simulink model "husky_sim - Copy"  (R2019b)
settings: Solver=ode4  StartTime=0.0  StopTime=3  FixedStep=0.006  RelTol=1e-3
InitFcn:
  | init_model;
values from neighbouring files (symbols this model uses):
  m = getfield(leg,'mass')    [dynamic_test.m]    (also in pen_init.m = link2.mass; test.mat = 2.2337)
  q_BL_K0 = initial_angle(12)    [func_params_ext.m]
  q_BR_K0 = initial_angle(9)    [func_params_ext.m]
  q_FL_K0 = initial_angle(6)    [func_params_ext.m]
undefined symbols (not defined in the file or in its folder): body, femur_left, femur_right, hip_left, hip_right, link_left, link_right, tarsus_left, tarsus_right, tibia_left, tibia_right, X, Y, Z
libraries: sm_lib x206, nesl_utility x56, dspsigops x7, Contact_Forces_Lib x4, simulink x2
(part 5 of 6)

== system husky_sim - Copy/Husky_simulator/robot_body/Leg_RL/tibia_rl ==
  Inertia : sm_lib/Body Elements/Inertia  InertiaType=Custom  Mass=tibia_left.mass  MassUnits=kg  CenterOfMass=[0, 0, 0]  CenterOfMassUnits=m  MomentsOfInertia=tibia_left.MomentsofInertia  MomentsOfInertiaUnits=kg*m^2  ProductsOfInertia=tibia_left.ProductsofInertia  ProductsOfInertiaUnits=kg*m^2  GraphicType=None  MarkerShape=Inertia  MarkerSize=20  GraphicVisPropType=SimpleVisualProperties  GraphicDiffuseColor=[0.5 0.5 0.5]  GraphicSpecularColor=[0.5 0.5 0.5 1.0]  GraphicAmbientColor=[0.15 0.15 0.15 1.0]  GraphicEmissiveColor=[0.0 0.0 0.0 1.0]  GraphicShininess=75  GraphicOpacity=1.0
  InertiaOriginTransform : sm_lib/Frames and Transforms/Rigid Transform  TranslationMethod=Cartesian  TranslationStandardOffset=0  TranslationLengthUnit=m  TranslationStandardAxis=+Z  TranslationCartesianOffset=[-0.10575, 0.0039831, 1.084e-05]  TranslationROffset=0  TranslationROffsetUnits=m  TranslationZOffset=0  TranslationZOffsetUnits=m  TranslationThetaOffset=0  TranslationThetaOffsetUnits=deg  RotationMethod=RotationSequence  RotationAngleUnits=deg  RotationStandardAxis=+Z  RotationAngle=0.0  RotationArbitraryAxis=[0 0 1]  FollAlignAxisA=+X  BaseAlignAxisA=+Y  FollAlignAxisB=+Y  BaseAlignAxisB=+Z  RotationSequenceAxes=BaseAxes  RotationSequence=XYZ  RotationSequenceAngles=[0, 0, 0]  RotationSequenceAnglesUnits=rad  RotationMatrix=[1 0 0; 0 1 0; 0 0 1]
  ReferenceFrame : sm_lib/Frames and Transforms/Reference Frame
  Visual : sm_lib/Body Elements/File Solid  ExtGeomFileName=husky/meshes/tibia_rl.STL  UnitType=Custom  ExtGeomFileUnits=m  StepReaderType=HEX  ExportEntireGeometry=off  InertiaType=Custom  Mass=0  MassUnits=kg  CenterOfMass=[0, 0, 0]  CenterOfMassUnits=m  MomentsOfInertia=[0, 0, 0]  MomentsOfInertiaUnits=kg*m^2  ProductsOfInertia=[0, 0, 0]  ProductsOfInertiaUnits=kg*m^2  BasedOnType=DensityFromFile  Density=1000  DensityUnits=kg/m^3  DoExposeReferenceFrame=on  SerializedFrames=<Frames/>  GraphicType=FromGeometry  MarkerShape=Sphere  MarkerSize=10  GraphicVisPropType=SimpleVisualProperties  GraphicDiffuseColor=[0, 0, 1]  GraphicSpecularColor=[0.5 0.5 0.5 1.0]  GraphicAmbientColor=[0.15 0.15 0.15 1.0]  GraphicEmissiveColor=[0.0 0.0 0.0 1.0]  GraphicShininess=75  GraphicOpacity=1
  VisualOriginTransform : sm_lib/Frames and Transforms/Rigid Transform  TranslationMethod=Cartesian  TranslationStandardOffset=0  TranslationLengthUnit=m  TranslationStandardAxis=+Z  TranslationCartesianOffset=[0, 0, 0]  TranslationROffset=0  TranslationROffsetUnits=m  TranslationZOffset=0  TranslationZOffsetUnits=m  TranslationThetaOffset=0  TranslationThetaOffsetUnits=deg  RotationMethod=RotationSequence  RotationAngleUnits=deg  RotationStandardAxis=+Z  RotationAngle=0.0  RotationArbitraryAxis=[0 0 1]  FollAlignAxisA=+X  BaseAlignAxisA=+Y  FollAlignAxisB=+Y  BaseAlignAxisB=+Z  RotationSequenceAxes=BaseAxes  RotationSequence=XYZ  RotationSequenceAngles=[0, 0, 0]  RotationSequenceAnglesUnits=rad  RotationMatrix=[1 0 0; 0 1 0; 0 0 1]
  ankle_rl_AxisTransform : sm_lib/Frames and Transforms/Rigid Transform  TranslationMethod=Cartesian  TranslationStandardOffset=0  TranslationLengthUnit=m  TranslationStandardAxis=+Z  TranslationCartesianOffset=[0, 0, 0]  TranslationROffset=0  TranslationROffsetUnits=m  TranslationZOffset=0  TranslationZOffsetUnits=m  TranslationThetaOffset=0  TranslationThetaOffsetUnits=deg  RotationMethod=ArbitraryAxis  RotationAngleUnits=rad  RotationStandardAxis=+Z  RotationAngle=-1.570796326794897  RotationArbitraryAxis=[-1, 0, 0]  FollAlignAxisA=+X  BaseAlignAxisA=+Y  FollAlignAxisB=+Y  BaseAlignAxisB=+Z  RotationSequenceAxes=FollowerAxes  RotationSequence=XYX  RotationSequenceAngles=[0 0 0]  RotationSequenceAnglesUnits=deg  RotationMatrix=[1 0 0; 0 1 0; 0 0 1]
  ankle_rl_OriginTransform : sm_lib/Frames and Transforms/Rigid Transform  TranslationMethod=Cartesian  TranslationStandardOffset=0  TranslationLengthUnit=m  TranslationStandardAxis=+Z  TranslationCartesianOffset=[-0.333, 0.0075, 0]  TranslationROffset=0  TranslationROffsetUnits=m  TranslationZOffset=0  TranslationZOffsetUnits=m  TranslationThetaOffset=0  TranslationThetaOffsetUnits=deg  RotationMethod=RotationSequence  RotationAngleUnits=deg  RotationStandardAxis=+Z  RotationAngle=0.0  RotationArbitraryAxis=[0 0 1]  FollAlignAxisA=+X  BaseAlignAxisA=+Y  FollAlignAxisB=+Y  BaseAlignAxisB=+Z  RotationSequenceAxes=BaseAxes  RotationSequence=XYZ  RotationSequenceAngles=[0, 0, 0]  RotationSequenceAnglesUnits=rad  RotationMatrix=[1 0 0; 0 1 0; 0 0 1]
  knee_rl_AxisInvTransform : sm_lib/Frames and Transforms/Rigid Transform  TranslationMethod=Cartesian  TranslationStandardOffset=0  TranslationLengthUnit=m  TranslationStandardAxis=+Z  TranslationCartesianOffset=[0, 0, 0]  TranslationROffset=0  TranslationROffsetUnits=m  TranslationZOffset=0  TranslationZOffsetUnits=m  TranslationThetaOffset=0  TranslationThetaOffsetUnits=deg  RotationMethod=ArbitraryAxis  RotationAngleUnits=rad  RotationStandardAxis=+Z  RotationAngle=1.570796326794897  RotationArbitraryAxis=[1, 0, 0]  FollAlignAxisA=+X  BaseAlignAxisA=+Y  FollAlignAxisB=+Y  BaseAlignAxisB=+Z  RotationSequenceAxes=FollowerAxes  RotationSequence=XYX  RotationSequenceAngles=[0 0 0]  RotationSequenceAnglesUnits=deg  RotationMatrix=[1 0 0; 0 1 0; 0 0 1]
  F : PMIOPort  Side=Left
  F1 : PMIOPort  Port=2  Side=Right
  connections:
  Inertia/RConn1 -- InertiaOriginTransform/RConn1
  ankle_rl_OriginTransform/LConn1 -- knee_rl_AxisInvTransform/LConn1 -- InertiaOriginTransform/LConn1 -- ReferenceFrame/RConn1 -- VisualOriginTransform/LConn1
  Visual/RConn1 -- VisualOriginTransform/RConn1
  ankle_rl_AxisTransform/RConn1 -- F1/RConn1
  ankle_rl_AxisTransform/LConn1 -- ankle_rl_OriginTransform/RConn1
  knee_rl_AxisInvTransform/RConn1 -- F/RConn1

== system husky_sim - Copy/Husky_simulator/robot_body/Leg_RR/femur_rr ==
  Inertia : sm_lib/Body Elements/Inertia  InertiaType=Custom  Mass=femur_right.mass  MassUnits=kg  CenterOfMass=[0, 0, 0]  CenterOfMassUnits=m  MomentsOfInertia=femur_right.MomentsofInertia  MomentsOfInertiaUnits=kg*m^2  ProductsOfInertia=femur_right.ProductsofInertia  ProductsOfInertiaUnits=kg*m^2  GraphicType=None  MarkerShape=Inertia  MarkerSize=20  GraphicVisPropType=SimpleVisualProperties  GraphicDiffuseColor=[0.5 0.5 0.5]  GraphicSpecularColor=[0.5 0.5 0.5 1.0]  GraphicAmbientColor=[0.15 0.15 0.15 1.0]  GraphicEmissiveColor=[0.0 0.0 0.0 1.0]  GraphicShininess=75  GraphicOpacity=1.0
  InertiaOriginTransform : sm_lib/Frames and Transforms/Rigid Transform  TranslationMethod=Cartesian  TranslationStandardOffset=0  TranslationLengthUnit=m  TranslationStandardAxis=+Z  TranslationCartesianOffset=[2.704e-07, -0.036112, -0.082829]  TranslationROffset=0  TranslationROffsetUnits=m  TranslationZOffset=0  TranslationZOffsetUnits=m  TranslationThetaOffset=0  TranslationThetaOffsetUnits=deg  RotationMethod=RotationSequence  RotationAngleUnits=deg  RotationStandardAxis=+Z  RotationAngle=0.0  RotationArbitraryAxis=[0 0 1]  FollAlignAxisA=+X  BaseAlignAxisA=+Y  FollAlignAxisB=+Y  BaseAlignAxisB=+Z  RotationSequenceAxes=BaseAxes  RotationSequence=XYZ  RotationSequenceAngles=[0, 0, 0]  RotationSequenceAnglesUnits=rad  RotationMatrix=[1 0 0; 0 1 0; 0 0 1]
  ReferenceFrame : sm_lib/Frames and Transforms/Reference Frame
  Visual : sm_lib/Body Elements/File Solid  ExtGeomFileName=husky/meshes/femur_rr.STL  UnitType=Custom  ExtGeomFileUnits=m  StepReaderType=HEX  ExportEntireGeometry=off  InertiaType=Custom  Mass=0  MassUnits=kg  CenterOfMass=[0, 0, 0]  CenterOfMassUnits=m  MomentsOfInertia=[0, 0, 0]  MomentsOfInertiaUnits=kg*m^2  ProductsOfInertia=[0, 0, 0]  ProductsOfInertiaUnits=kg*m^2  BasedOnType=DensityFromFile  Density=1000  DensityUnits=kg/m^3  DoExposeReferenceFrame=on  SerializedFrames=<Frames/>  GraphicType=FromGeometry  MarkerShape=Sphere  MarkerSize=10  GraphicVisPropType=SimpleVisualProperties  GraphicDiffuseColor=[0, 1, 0]  GraphicSpecularColor=[0.5 0.5 0.5 1.0]  GraphicAmbientColor=[0.15 0.15 0.15 1.0]  GraphicEmissiveColor=[0.0 0.0 0.0 1.0]  GraphicShininess=75  GraphicOpacity=1
  VisualOriginTransform : sm_lib/Frames and Transforms/Rigid Transform  TranslationMethod=Cartesian  TranslationStandardOffset=0  TranslationLengthUnit=m  TranslationStandardAxis=+Z  TranslationCartesianOffset=[0, 0, 0]  TranslationROffset=0  TranslationROffsetUnits=m  TranslationZOffset=0  TranslationZOffsetUnits=m  TranslationThetaOffset=0  TranslationThetaOffsetUnits=deg  RotationMethod=RotationSequence  RotationAngleUnits=deg  RotationStandardAxis=+Z  RotationAngle=0.0  RotationArbitraryAxis=[0 0 1]  FollAlignAxisA=+X  BaseAlignAxisA=+Y  FollAlignAxisB=+Y  BaseAlignAxisB=+Z  RotationSequenceAxes=BaseAxes  RotationSequence=XYZ  RotationSequenceAngles=[0, 0, 0]  RotationSequenceAnglesUnits=rad  RotationMatrix=[1 0 0; 0 1 0; 0 0 1]
  hip_rr_ex_AxisInvTransform : sm_lib/Frames and Transforms/Rigid Transform  TranslationMethod=Cartesian  TranslationStandardOffset=0  TranslationLengthUnit=m  TranslationStandardAxis=+Z  TranslationCartesianOffset=[0, 0, 0]  TranslationROffset=0  TranslationROffsetUnits=m  TranslationZOffset=0  TranslationZOffsetUnits=m  TranslationThetaOffset=0  TranslationThetaOffsetUnits=deg  RotationMethod=ArbitraryAxis  RotationAngleUnits=rad  RotationStandardAxis=+Z  RotationAngle=1.570796326794897  RotationArbitraryAxis=[1, 0, 0]  FollAlignAxisA=+X  BaseAlignAxisA=+Y  FollAlignAxisB=+Y  BaseAlignAxisB=+Z  RotationSequenceAxes=FollowerAxes  RotationSequence=XYX  RotationSequenceAngles=[0 0 0]  RotationSequenceAnglesUnits=deg  RotationMatrix=[1 0 0; 0 1 0; 0 0 1]
  knee_rr_AxisTransform : sm_lib/Frames and Transforms/Rigid Transform  TranslationMethod=Cartesian  TranslationStandardOffset=0  TranslationLengthUnit=m  TranslationStandardAxis=+Z  TranslationCartesianOffset=[0, 0, 0]  TranslationROffset=0  TranslationROffsetUnits=m  TranslationZOffset=0  TranslationZOffsetUnits=m  TranslationThetaOffset=0  TranslationThetaOffsetUnits=deg  RotationMethod=ArbitraryAxis  RotationAngleUnits=rad  RotationStandardAxis=+Z  RotationAngle=1.570796326794897  RotationArbitraryAxis=[-1, 0, 0]  FollAlignAxisA=+X  BaseAlignAxisA=+Y  FollAlignAxisB=+Y  BaseAlignAxisB=+Z  RotationSequenceAxes=FollowerAxes  RotationSequence=XYX  RotationSequenceAngles=[0 0 0]  RotationSequenceAnglesUnits=deg  RotationMatrix=[1 0 0; 0 1 0; 0 0 1]
  knee_rr_OriginTransform : sm_lib/Frames and Transforms/Rigid Transform  TranslationMethod=Cartesian  TranslationStandardOffset=0  TranslationLengthUnit=m  TranslationStandardAxis=+Z  TranslationCartesianOffset=[0, 0, -0.158]  TranslationROffset=0  TranslationROffsetUnits=m  TranslationZOffset=0  TranslationZOffsetUnits=m  TranslationThetaOffset=0  TranslationThetaOffsetUnits=deg  RotationMethod=RotationSequence  RotationAngleUnits=deg  RotationStandardAxis=+Z  RotationAngle=0.0  RotationArbitraryAxis=[0 0 1]  FollAlignAxisA=+X  BaseAlignAxisA=+Y  FollAlignAxisB=+Y  BaseAlignAxisB=+Z  RotationSequenceAxes=BaseAxes  RotationSequence=XYZ  RotationSequenceAngles=[0, 0, 0]  RotationSequenceAnglesUnits=rad  RotationMatrix=[1 0 0; 0 1 0; 0 0 1]
  F : PMIOPort  Side=Left
  F1 : PMIOPort  Port=2  Side=Right
  connections:
  Inertia/RConn1 -- InertiaOriginTransform/RConn1
  InertiaOriginTransform/LConn1 -- hip_rr_ex_AxisInvTransform/LConn1 -- knee_rr_OriginTransform/LConn1 -- VisualOriginTransform/LConn1 -- ReferenceFrame/RConn1
  Visual/RConn1 -- VisualOriginTransform/RConn1
  hip_rr_ex_AxisInvTransform/RConn1 -- F/RConn1
  knee_rr_AxisTransform/RConn1 -- F1/RConn1
  knee_rr_AxisTransform/LConn1 -- knee_rr_OriginTransform/RConn1

== system husky_sim - Copy/Husky_simulator/robot_body/Leg_RR/hip_rr ==
  Inertia : sm_lib/Body Elements/Inertia  InertiaType=Custom  Mass=hip_right.mass  MassUnits=kg  CenterOfMass=[0,0,0]  CenterOfMassUnits=m  MomentsOfInertia=hip_right.MomentsofInertia  MomentsOfInertiaUnits=kg*m^2  ProductsOfInertia=hip_right.ProductsofInertia  ProductsOfInertiaUnits=kg*m^2  GraphicType=None  MarkerShape=Inertia  MarkerSize=20  GraphicVisPropType=SimpleVisualProperties  GraphicDiffuseColor=[0.5 0.5 0.5]  GraphicSpecularColor=[0.5 0.5 0.5 1.0]  GraphicAmbientColor=[0.15 0.15 0.15 1.0]  GraphicEmissiveColor=[0.0 0.0 0.0 1.0]  GraphicShininess=75  GraphicOpacity=1.0
  InertiaOriginTransform : sm_lib/Frames and Transforms/Rigid Transform  TranslationMethod=Cartesian  TranslationStandardOffset=0  TranslationLengthUnit=m  TranslationStandardAxis=+Z  TranslationCartesianOffset=[0.024751, 0.0025459, 6.0284e-05]  TranslationROffset=0  TranslationROffsetUnits=m  TranslationZOffset=0  TranslationZOffsetUnits=m  TranslationThetaOffset=0  TranslationThetaOffsetUnits=deg  RotationMethod=RotationSequence  RotationAngleUnits=deg  RotationStandardAxis=+Z  RotationAngle=0.0  RotationArbitraryAxis=[0 0 1]  FollAlignAxisA=+X  BaseAlignAxisA=+Y  FollAlignAxisB=+Y  BaseAlignAxisB=+Z  RotationSequenceAxes=BaseAxes  RotationSequence=XYZ  RotationSequenceAngles=[0, 0, 0]  RotationSequenceAnglesUnits=rad  RotationMatrix=[1 0 0; 0 1 0; 0 0 1]
  ReferenceFrame : sm_lib/Frames and Transforms/Reference Frame
  Visual : sm_lib/Body Elements/File Solid  ExtGeomFileName=husky/meshes/hip_rr.STL  UnitType=Custom  ExtGeomFileUnits=m  StepReaderType=HEX  ExportEntireGeometry=off  InertiaType=Custom  Mass=0  MassUnits=kg  CenterOfMass=[0, 0, 0]  CenterOfMassUnits=m  MomentsOfInertia=[0, 0, 0]  MomentsOfInertiaUnits=kg*m^2  ProductsOfInertia=[0, 0, 0]  ProductsOfInertiaUnits=kg*m^2  BasedOnType=DensityFromFile  Density=1000  DensityUnits=kg/m^3  DoExposeReferenceFrame=on  SerializedFrames=<Frames/>  GraphicType=FromGeometry  MarkerShape=Sphere  MarkerSize=10  GraphicVisPropType=SimpleVisualProperties  GraphicDiffuseColor=[1, 0, 0]  GraphicSpecularColor=[0.5 0.5 0.5 1.0]  GraphicAmbientColor=[0.15 0.15 0.15 1.0]  GraphicEmissiveColor=[0.0 0.0 0.0 1.0]  GraphicShininess=75  GraphicOpacity=1
  VisualOriginTransform : sm_lib/Frames and Transforms/Rigid Transform  TranslationMethod=Cartesian  TranslationStandardOffset=0  TranslationLengthUnit=m  TranslationStandardAxis=+Z  TranslationCartesianOffset=[0, 0, 0]  TranslationROffset=0  TranslationROffsetUnits=m  TranslationZOffset=0  TranslationZOffsetUnits=m  TranslationThetaOffset=0  TranslationThetaOffsetUnits=deg  RotationMethod=RotationSequence  RotationAngleUnits=deg  RotationStandardAxis=+Z  RotationAngle=0.0  RotationArbitraryAxis=[0 0 1]  FollAlignAxisA=+X  BaseAlignAxisA=+Y  FollAlignAxisB=+Y  BaseAlignAxisB=+Z  RotationSequenceAxes=BaseAxes  RotationSequence=XYZ  RotationSequenceAngles=[0, 0, 0]  RotationSequenceAnglesUnits=rad  RotationMatrix=[1 0 0; 0 1 0; 0 0 1]
  hip_rr_ab_AxisInvTransform : sm_lib/Frames and Transforms/Rigid Transform  TranslationMethod=Cartesian  TranslationStandardOffset=0  TranslationLengthUnit=m  TranslationStandardAxis=+Z  TranslationCartesianOffset=[0, 0, 0]  TranslationROffset=0  TranslationROffsetUnits=m  TranslationZOffset=0  TranslationZOffsetUnits=m  TranslationThetaOffset=0  TranslationThetaOffsetUnits=deg  RotationMethod=ArbitraryAxis  RotationAngleUnits=rad  RotationStandardAxis=+Z  RotationAngle=1.570796326794897  RotationArbitraryAxis=[-0, -1, 0]  FollAlignAxisA=+X  BaseAlignAxisA=+Y  FollAlignAxisB=+Y  BaseAlignAxisB=+Z  RotationSequenceAxes=FollowerAxes  RotationSequence=XYX  RotationSequenceAngles=[0 0 0]  RotationSequenceAnglesUnits=deg  RotationMatrix=[1 0 0; 0 1 0; 0 0 1]
  hip_rr_ex_AxisTransform : sm_lib/Frames and Transforms/Rigid Transform  TranslationMethod=Cartesian  TranslationStandardOffset=0  TranslationLengthUnit=m  TranslationStandardAxis=+Z  TranslationCartesianOffset=[0, 0, 0]  TranslationROffset=0  TranslationROffsetUnits=m  TranslationZOffset=0  TranslationZOffsetUnits=m  TranslationThetaOffset=0  TranslationThetaOffsetUnits=deg  RotationMethod=ArbitraryAxis  RotationAngleUnits=rad  RotationStandardAxis=+Z  RotationAngle=1.570796326794897  RotationArbitraryAxis=[1, 0, 0]  FollAlignAxisA=+X  BaseAlignAxisA=+Y  FollAlignAxisB=+Y  BaseAlignAxisB=+Z  RotationSequenceAxes=FollowerAxes  RotationSequence=XYX  RotationSequenceAngles=[0 0 0]  RotationSequenceAnglesUnits=deg  RotationMatrix=[1 0 0; 0 1 0; 0 0 1]
  hip_rr_ex_OriginTransform : sm_lib/Frames and Transforms/Rigid Transform  TranslationMethod=Cartesian  TranslationStandardOffset=0  TranslationLengthUnit=m  TranslationStandardAxis=+Z  TranslationCartesianOffset=[0.053, 0.007, 0]  TranslationROffset=0  TranslationROffsetUnits=m  TranslationZOffset=0  TranslationZOffsetUnits=m  TranslationThetaOffset=0  TranslationThetaOffsetUnits=deg  RotationMethod=RotationSequence  RotationAngleUnits=deg  RotationStandardAxis=+Z  RotationAngle=0.0  RotationArbitraryAxis=[0 0 1]  FollAlignAxisA=+X  BaseAlignAxisA=+Y  FollAlignAxisB=+Y  BaseAlignAxisB=+Z  RotationSequenceAxes=BaseAxes  RotationSequence=XYZ  RotationSequenceAngles=[0, 0, 0]  RotationSequenceAnglesUnits=rad  RotationMatrix=[1 0 0; 0 1 0; 0 0 1]
  F : PMIOPort  Side=Left
  F1 : PMIOPort  Port=2  Side=Right
  connections:
  Inertia/RConn1 -- InertiaOriginTransform/RConn1
  hip_rr_ab_AxisInvTransform/LConn1 -- hip_rr_ex_OriginTransform/LConn1 -- InertiaOriginTransform/LConn1 -- ReferenceFrame/RConn1 -- VisualOriginTransform/LConn1
  Visual/RConn1 -- VisualOriginTransform/RConn1
  hip_rr_ab_AxisInvTransform/RConn1 -- F/RConn1
  hip_rr_ex_AxisTransform/RConn1 -- F1/RConn1
  hip_rr_ex_AxisTransform/LConn1 -- hip_rr_ex_OriginTransform/RConn1

== system husky_sim - Copy/Husky_simulator/robot_body/Leg_RR/link_rr ==
  Inertia : sm_lib/Body Elements/Inertia  InertiaType=Custom  Mass=link_right.mass  MassUnits=kg  CenterOfMass=[0, 0, 0]  CenterOfMassUnits=m  MomentsOfInertia=link_right.MomentsofInertia  MomentsOfInertiaUnits=kg*m^2  ProductsOfInertia=link_right.ProductsofInertia  ProductsOfInertiaUnits=kg*m^2  GraphicType=None  MarkerShape=Inertia  MarkerSize=20  GraphicVisPropType=SimpleVisualProperties  GraphicDiffuseColor=[0.5 0.5 0.5]  GraphicSpecularColor=[0.5 0.5 0.5 1.0]  GraphicAmbientColor=[0.15 0.15 0.15 1.0]  GraphicEmissiveColor=[0.0 0.0 0.0 1.0]  GraphicShininess=75  GraphicOpacity=1.0
  InertiaOriginTransform : sm_lib/Frames and Transforms/Rigid Transform  TranslationMethod=Cartesian  TranslationStandardOffset=0  TranslationLengthUnit=m  TranslationStandardAxis=+Z  TranslationCartesianOffset=[0.15598, -0.09087199999999999, -1.3564e-10]  TranslationROffset=0  TranslationROffsetUnits=m  TranslationZOffset=0  TranslationZOffsetUnits=m  TranslationThetaOffset=0  TranslationThetaOffsetUnits=deg  RotationMethod=RotationSequence  RotationAngleUnits=deg  RotationStandardAxis=+Z  RotationAngle=0.0  RotationArbitraryAxis=[0 0 1]  FollAlignAxisA=+X  BaseAlignAxisA=+Y  FollAlignAxisB=+Y  BaseAlignAxisB=+Z  RotationSequenceAxes=BaseAxes  RotationSequence=XYZ  RotationSequenceAngles=[0, 0, 0]  RotationSequenceAnglesUnits=rad  RotationMatrix=[1 0 0; 0 1 0; 0 0 1]
  ReferenceFrame : sm_lib/Frames and Transforms/Reference Frame
  Visual : sm_lib/Body Elements/File Solid  ExtGeomFileName=husky/meshes/link_rr.STL  UnitType=Custom  ExtGeomFileUnits=m  StepReaderType=HEX  ExportEntireGeometry=off  InertiaType=Custom  Mass=0  MassUnits=kg  CenterOfMass=[0, 0, 0]  CenterOfMassUnits=m  MomentsOfInertia=[0, 0, 0]  MomentsOfInertiaUnits=kg*m^2  ProductsOfInertia=[0, 0, 0]  ProductsOfInertiaUnits=kg*m^2  BasedOnType=DensityFromFile  Density=1000  DensityUnits=kg/m^3  DoExposeReferenceFrame=on  SerializedFrames=<Frames/>  GraphicType=FromGeometry  MarkerShape=Sphere  MarkerSize=10  GraphicVisPropType=SimpleVisualProperties  GraphicDiffuseColor=[1, 0, 0.5]  GraphicSpecularColor=[0.5 0.5 0.5 1.0]  GraphicAmbientColor=[0.15 0.15 0.15 1.0]  GraphicEmissiveColor=[0.0 0.0 0.0 1.0]  GraphicShininess=75  GraphicOpacity=1
  VisualOriginTransform : sm_lib/Frames and Transforms/Rigid Transform  TranslationMethod=Cartesian  TranslationStandardOffset=0  TranslationLengthUnit=m  TranslationStandardAxis=+Z  TranslationCartesianOffset=[0, 0, 0]  TranslationROffset=0  TranslationROffsetUnits=m  TranslationZOffset=0  TranslationZOffsetUnits=m  TranslationThetaOffset=0  TranslationThetaOffsetUnits=deg  RotationMethod=RotationSequence  RotationAngleUnits=deg  RotationStandardAxis=+Z  RotationAngle=0.0  RotationArbitraryAxis=[0 0 1]  FollAlignAxisA=+X  BaseAlignAxisA=+Y  FollAlignAxisB=+Y  BaseAlignAxisB=+Z  RotationSequenceAxes=BaseAxes  RotationSequence=XYZ  RotationSequenceAngles=[0, 0, 0]  RotationSequenceAnglesUnits=rad  RotationMatrix=[1 0 0; 0 1 0; 0 0 1]
  link1_rr_AxisInvTransform : sm_lib/Frames and Transforms/Rigid Transform  TranslationMethod=Cartesian  TranslationStandardOffset=0  TranslationLengthUnit=m  TranslationStandardAxis=+Z  TranslationCartesianOffset=[0, 0, 0]  TranslationROffset=0  TranslationROffsetUnits=m  TranslationZOffset=0  TranslationZOffsetUnits=m  TranslationThetaOffset=0  TranslationThetaOffsetUnits=deg  RotationMethod=ArbitraryAxis  RotationAngleUnits=rad  RotationStandardAxis=+Z  RotationAngle=1.570796326794897  RotationArbitraryAxis=[1, 0, 0]  FollAlignAxisA=+X  BaseAlignAxisA=+Y  FollAlignAxisB=+Y  BaseAlignAxisB=+Z  RotationSequenceAxes=FollowerAxes  RotationSequence=XYX  RotationSequenceAngles=[0 0 0]  RotationSequenceAnglesUnits=deg  RotationMatrix=[1 0 0; 0 1 0; 0 0 1]
  F : PMIOPort  Side=Left
  connections:
  Inertia/RConn1 -- InertiaOriginTransform/RConn1
  InertiaOriginTransform/LConn1 -- VisualOriginTransform/LConn1 -- link1_rr_AxisInvTransform/LConn1 -- ReferenceFrame/RConn1
  Visual/RConn1 -- VisualOriginTransform/RConn1
  link1_rr_AxisInvTransform/RConn1 -- F/RConn1

== system husky_sim - Copy/Husky_simulator/robot_body/Leg_RR/tarsus_rr  ==
  Inertia : sm_lib/Body Elements/Inertia  InertiaType=Custom  Mass=tarsus_right.mass  MassUnits=kg  CenterOfMass=[0, 0, 0]  CenterOfMassUnits=m  MomentsOfInertia=tarsus_right.MomentsofInertia  MomentsOfInertiaUnits=kg*m^2  ProductsOfInertia=tarsus_right.ProductsofInertia  ProductsOfInertiaUnits=kg*m^2  GraphicType=None  MarkerShape=Inertia  MarkerSize=20  GraphicVisPropType=SimpleVisualProperties  GraphicDiffuseColor=[0.5 0.5 0.5]  GraphicSpecularColor=[0.5 0.5 0.5 1.0]  GraphicAmbientColor=[0.15 0.15 0.15 1.0]  GraphicEmissiveColor=[0.0 0.0 0.0 1.0]  GraphicShininess=75  GraphicOpacity=1.0
  InertiaOriginTransform : sm_lib/Frames and Transforms/Rigid Transform  TranslationMethod=Cartesian  TranslationStandardOffset=0  TranslationLengthUnit=m  TranslationStandardAxis=+Z  TranslationCartesianOffset=[-3.6453e-11, -2.4587e-10, -0.054555]  TranslationROffset=0  TranslationROffsetUnits=m  TranslationZOffset=0  TranslationZOffsetUnits=m  TranslationThetaOffset=0  TranslationThetaOffsetUnits=deg  RotationMethod=RotationSequence  RotationAngleUnits=deg  RotationStandardAxis=+Z  RotationAngle=0.0  RotationArbitraryAxis=[0 0 1]  FollAlignAxisA=+X  BaseAlignAxisA=+Y  FollAlignAxisB=+Y  BaseAlignAxisB=+Z  RotationSequenceAxes=BaseAxes  RotationSequence=XYZ  RotationSequenceAngles=[0, 0, 0]  RotationSequenceAnglesUnits=rad  RotationMatrix=[1 0 0; 0 1 0; 0 0 1]
  ReferenceFrame : sm_lib/Frames and Transforms/Reference Frame
  Visual : sm_lib/Body Elements/File Solid  ExtGeomFileName=husky/meshes/tarsus_rr.STL  UnitType=Custom  ExtGeomFileUnits=m  StepReaderType=HEX  ExportEntireGeometry=off  InertiaType=Custom  Mass=0  MassUnits=kg  CenterOfMass=[0, 0, 0]  CenterOfMassUnits=m  MomentsOfInertia=[0, 0, 0]  MomentsOfInertiaUnits=kg*m^2  ProductsOfInertia=[0, 0, 0]  ProductsOfInertiaUnits=kg*m^2  BasedOnType=DensityFromFile  Density=1000  DensityUnits=kg/m^3  DoExposeReferenceFrame=on  SerializedFrames=<Frames/>  GraphicType=FromGeometry  MarkerShape=Sphere  MarkerSize=10  GraphicVisPropType=SimpleVisualProperties  GraphicDiffuseColor=[0.6 1.0 1.0]  GraphicSpecularColor=[0.5 0.5 0.5 1.0]  GraphicAmbientColor=[0.15 0.15 0.15 1.0]  GraphicEmissiveColor=[0.0 0.0 0.0 1.0]  GraphicShininess=75  GraphicOpacity=1
  VisualOriginTransform : sm_lib/Frames and Transforms/Rigid Transform  TranslationMethod=Cartesian  TranslationStandardOffset=0  TranslationLengthUnit=m  TranslationStandardAxis=+Z  TranslationCartesianOffset=[0, 0, 0]  TranslationROffset=0  TranslationROffsetUnits=m  TranslationZOffset=0  TranslationZOffsetUnits=m  TranslationThetaOffset=0  TranslationThetaOffsetUnits=deg  RotationMethod=RotationSequence  RotationAngleUnits=deg  RotationStandardAxis=+Z  RotationAngle=0.0  RotationArbitraryAxis=[0 0 1]  FollAlignAxisA=+X  BaseAlignAxisA=+Y  FollAlignAxisB=+Y  BaseAlignAxisB=+Z  RotationSequenceAxes=BaseAxes  RotationSequence=XYZ  RotationSequenceAngles=[0, 0, 0]  RotationSequenceAnglesUnits=rad  RotationMatrix=[1 0 0; 0 1 0; 0 0 1]
  ankle_rr_AxisInvTransform : sm_lib/Frames and Transforms/Rigid Transform  TranslationMethod=Cartesian  TranslationStandardOffset=0  TranslationLengthUnit=m  TranslationStandardAxis=+Z  TranslationCartesianOffset=[0, 0, 0]  TranslationROffset=0  TranslationROffsetUnits=m  TranslationZOffset=0  TranslationZOffsetUnits=m  TranslationThetaOffset=0  TranslationThetaOffsetUnits=deg  RotationMethod=ArbitraryAxis  RotationAngleUnits=rad  RotationStandardAxis=+Z  RotationAngle=1.570796326794897  RotationArbitraryAxis=[-1, 0, 0]  FollAlignAxisA=+X  BaseAlignAxisA=+Y  FollAlignAxisB=+Y  BaseAlignAxisB=+Z  RotationSequenceAxes=FollowerAxes  RotationSequence=XYX  RotationSequenceAngles=[0 0 0]  RotationSequenceAnglesUnits=deg  RotationMatrix=[1 0 0; 0 1 0; 0 0 1]
  foot_contact : sm_lib/Frames and Transforms/Rigid Transform  TranslationMethod=Cartesian  TranslationStandardOffset=0  TranslationLengthUnit=m  TranslationStandardAxis=+Z  TranslationCartesianOffset=[0 0 -0.120]  TranslationROffset=0  TranslationROffsetUnits=m  TranslationZOffset=0  TranslationZOffsetUnits=m  TranslationThetaOffset=0  TranslationThetaOffsetUnits=deg  RotationMethod=RotationSequence  RotationAngleUnits=deg  RotationStandardAxis=+Z  RotationAngle=0.0  RotationArbitraryAxis=[0 0 1]  FollAlignAxisA=+X  BaseAlignAxisA=+Y  FollAlignAxisB=+Y  BaseAlignAxisB=+Z  RotationSequenceAxes=BaseAxes  RotationSequence=XYZ  RotationSequenceAngles=[0, 0, 0]  RotationSequenceAnglesUnits=rad  RotationMatrix=[1 0 0; 0 1 0; 0 0 1]
  link1_rr_AxisTransform : sm_lib/Frames and Transforms/Rigid Transform  TranslationMethod=Cartesian  TranslationStandardOffset=0  TranslationLengthUnit=m  TranslationStandardAxis=+Z  TranslationCartesianOffset=[0, 0, 0]  TranslationROffset=0  TranslationROffsetUnits=m  TranslationZOffset=0  TranslationZOffsetUnits=m  TranslationThetaOffset=0  TranslationThetaOffsetUnits=deg  RotationMethod=ArbitraryAxis  RotationAngleUnits=rad  RotationStandardAxis=+Z  RotationAngle=1.570796326794897  RotationArbitraryAxis=[1, 0, 0]  FollAlignAxisA=+X  BaseAlignAxisA=+Y  FollAlignAxisB=+Y  BaseAlignAxisB=+Z  RotationSequenceAxes=FollowerAxes  RotationSequence=XYX  RotationSequenceAngles=[0 0 0]  RotationSequenceAnglesUnits=deg  RotationMatrix=[1 0 0; 0 1 0; 0 0 1]
  link1_rr_OriginTransform : sm_lib/Frames and Transforms/Rigid Transform  TranslationMethod=Cartesian  TranslationStandardOffset=0  TranslationLengthUnit=m  TranslationStandardAxis=+Z  TranslationCartesianOffset=[0, 0.0910000000016747, 0.0600000000001059]  TranslationROffset=0  TranslationROffsetUnits=m  TranslationZOffset=0  TranslationZOffsetUnits=m  TranslationThetaOffset=0  TranslationThetaOffsetUnits=deg  RotationMethod=RotationSequence  RotationAngleUnits=deg  RotationStandardAxis=+Z  RotationAngle=0.0  RotationArbitraryAxis=[0 0 1]  FollAlignAxisA=+X  BaseAlignAxisA=+Y  FollAlignAxisB=+Y  BaseAlignAxisB=+Z  RotationSequenceAxes=BaseAxes  RotationSequence=XYZ  RotationSequenceAngles=[0, 0, 0]  RotationSequenceAnglesUnits=rad  RotationMatrix=[1 0 0; 0 1 0; 0 0 1]
  F : PMIOPort  Side=Left
  F2 : PMIOPort  Port=2  Side=Right
  link : PMIOPort  Port=3  Side=Right
  connections:
  Inertia/RConn1 -- InertiaOriginTransform/RConn1
  ankle_rr_AxisInvTransform/LConn1 -- link1_rr_OriginTransform/LConn1 -- foot_contact/LConn1 -- VisualOriginTransform/LConn1 -- InertiaOriginTransform/LConn1 -- ReferenceFrame/RConn1
  Visual/RConn1 -- VisualOriginTransform/RConn1
  ankle_rr_AxisInvTransform/RConn1 -- F/RConn1
  F2/RConn1 -- foot_contact/RConn1
  link1_rr_AxisTransform/RConn1 -- link/RConn1
  link1_rr_AxisTransform/LConn1 -- link1_rr_OriginTransform/RConn1

== system husky_sim - Copy/Husky_simulator/robot_body/Leg_RR/tibia_rr ==
  Inertia : sm_lib/Body Elements/Inertia  InertiaType=Custom  Mass=tibia_right.mass  MassUnits=kg  CenterOfMass=[0, 0, 0]  CenterOfMassUnits=m  MomentsOfInertia=tibia_right.MomentsofInertia  MomentsOfInertiaUnits=kg*m^2  ProductsOfInertia=tibia_right.ProductsofInertia  ProductsOfInertiaUnits=kg*m^2  GraphicType=None  MarkerShape=Inertia  MarkerSize=20  GraphicVisPropType=SimpleVisualProperties  GraphicDiffuseColor=[0.5 0.5 0.5]  GraphicSpecularColor=[0.5 0.5 0.5 1.0]  GraphicAmbientColor=[0.15 0.15 0.15 1.0]  GraphicEmissiveColor=[0.0 0.0 0.0 1.0]  GraphicShininess=75  GraphicOpacity=1.0
  InertiaOriginTransform : sm_lib/Frames and Transforms/Rigid Transform  TranslationMethod=Cartesian  TranslationStandardOffset=0  TranslationLengthUnit=m  TranslationStandardAxis=+Z  TranslationCartesianOffset=[-0.10575, -0.0039831, -1.084e-05]  TranslationROffset=0  TranslationROffsetUnits=m  TranslationZOffset=0  TranslationZOffsetUnits=m  TranslationThetaOffset=0  TranslationThetaOffsetUnits=deg  RotationMethod=RotationSequence  RotationAngleUnits=deg  RotationStandardAxis=+Z  RotationAngle=0.0  RotationArbitraryAxis=[0 0 1]  FollAlignAxisA=+X  BaseAlignAxisA=+Y  FollAlignAxisB=+Y  BaseAlignAxisB=+Z  RotationSequenceAxes=BaseAxes  RotationSequence=XYZ  RotationSequenceAngles=[0, 0, 0]  RotationSequenceAnglesUnits=rad  RotationMatrix=[1 0 0; 0 1 0; 0 0 1]
  ReferenceFrame : sm_lib/Frames and Transforms/Reference Frame
  Visual : sm_lib/Body Elements/File Solid  ExtGeomFileName=husky/meshes/tibia_rr.STL  UnitType=Custom  ExtGeomFileUnits=m  StepReaderType=HEX  ExportEntireGeometry=off  InertiaType=Custom  Mass=0  MassUnits=kg  CenterOfMass=[0, 0, 0]  CenterOfMassUnits=m  MomentsOfInertia=[0, 0, 0]  MomentsOfInertiaUnits=kg*m^2  ProductsOfInertia=[0, 0, 0]  ProductsOfInertiaUnits=kg*m^2  BasedOnType=DensityFromFile  Density=1000  DensityUnits=kg/m^3  DoExposeReferenceFrame=on  SerializedFrames=<Frames/>  GraphicType=FromGeometry  MarkerShape=Sphere  MarkerSize=10  GraphicVisPropType=SimpleVisualProperties  GraphicDiffuseColor=[0, 0, 1]  GraphicSpecularColor=[0.5 0.5 0.5 1.0]  GraphicAmbientColor=[0.15 0.15 0.15 1.0]  GraphicEmissiveColor=[0.0 0.0 0.0 1.0]  GraphicShininess=75  GraphicOpacity=1
  VisualOriginTransform : sm_lib/Frames and Transforms/Rigid Transform  TranslationMethod=Cartesian  TranslationStandardOffset=0  TranslationLengthUnit=m  TranslationStandardAxis=+Z  TranslationCartesianOffset=[0, 0, 0]  TranslationROffset=0  TranslationROffsetUnits=m  TranslationZOffset=0  TranslationZOffsetUnits=m  TranslationThetaOffset=0  TranslationThetaOffsetUnits=deg  RotationMethod=RotationSequence  RotationAngleUnits=deg  RotationStandardAxis=+Z  RotationAngle=0.0  RotationArbitraryAxis=[0 0 1]  FollAlignAxisA=+X  BaseAlignAxisA=+Y  FollAlignAxisB=+Y  BaseAlignAxisB=+Z  RotationSequenceAxes=BaseAxes  RotationSequence=XYZ  RotationSequenceAngles=[0, 0, 0]  RotationSequenceAnglesUnits=rad  RotationMatrix=[1 0 0; 0 1 0; 0 0 1]
  ankle_rr_AxisTransform : sm_lib/Frames and Transforms/Rigid Transform  TranslationMethod=Cartesian  TranslationStandardOffset=0  TranslationLengthUnit=m  TranslationStandardAxis=+Z  TranslationCartesianOffset=[0, 0, 0]  TranslationROffset=0  TranslationROffsetUnits=m  TranslationZOffset=0  TranslationZOffsetUnits=m  TranslationThetaOffset=0  TranslationThetaOffsetUnits=deg  RotationMethod=ArbitraryAxis  RotationAngleUnits=rad  RotationStandardAxis=+Z  RotationAngle=1.570796326794897  RotationArbitraryAxis=[-1, 0, 0]  FollAlignAxisA=+X  BaseAlignAxisA=+Y  FollAlignAxisB=+Y  BaseAlignAxisB=+Z  RotationSequenceAxes=FollowerAxes  RotationSequence=XYX  RotationSequenceAngles=[0 0 0]  RotationSequenceAnglesUnits=deg  RotationMatrix=[1 0 0; 0 1 0; 0 0 1]
  ankle_rr_OriginTransform : sm_lib/Frames and Transforms/Rigid Transform  TranslationMethod=Cartesian  TranslationStandardOffset=0  TranslationLengthUnit=m  TranslationStandardAxis=+Z  TranslationCartesianOffset=[-0.333, -0.0075, 0]  TranslationROffset=0  TranslationROffsetUnits=m  TranslationZOffset=0  TranslationZOffsetUnits=m  TranslationThetaOffset=0  TranslationThetaOffsetUnits=deg  RotationMethod=RotationSequence  RotationAngleUnits=deg  RotationStandardAxis=+Z  RotationAngle=0.0  RotationArbitraryAxis=[0 0 1]  FollAlignAxisA=+X  BaseAlignAxisA=+Y  FollAlignAxisB=+Y  BaseAlignAxisB=+Z  RotationSequenceAxes=BaseAxes  RotationSequence=XYZ  RotationSequenceAngles=[0, 0, 0]  RotationSequenceAnglesUnits=rad  RotationMatrix=[1 0 0; 0 1 0; 0 0 1]
  knee_rr_AxisInvTransform : sm_lib/Frames and Transforms/Rigid Transform  TranslationMethod=Cartesian  TranslationStandardOffset=0  TranslationLengthUnit=m  TranslationStandardAxis=+Z  TranslationCartesianOffset=[0, 0, 0]  TranslationROffset=0  TranslationROffsetUnits=m  TranslationZOffset=0  TranslationZOffsetUnits=m  TranslationThetaOffset=0  TranslationThetaOffsetUnits=deg  RotationMethod=ArbitraryAxis  RotationAngleUnits=rad  RotationStandardAxis=+Z  RotationAngle=1.570796326794897  RotationArbitraryAxis=[-1, 0, 0]  FollAlignAxisA=+X  BaseAlignAxisA=+Y  FollAlignAxisB=+Y  BaseAlignAxisB=+Z  RotationSequenceAxes=FollowerAxes  RotationSequence=XYX  RotationSequenceAngles=[0 0 0]  RotationSequenceAnglesUnits=deg  RotationMatrix=[1 0 0; 0 1 0; 0 0 1]
  F : PMIOPort  Side=Left
  F1 : PMIOPort  Port=2  Side=Right
  connections:
  Inertia/RConn1 -- InertiaOriginTransform/RConn1
  InertiaOriginTransform/LConn1 -- ankle_rr_OriginTransform/LConn1 -- knee_rr_AxisInvTransform/LConn1 -- VisualOriginTransform/LConn1 -- ReferenceFrame/RConn1
  Visual/RConn1 -- VisualOriginTransform/RConn1
  ankle_rr_AxisTransform/RConn1 -- F1/RConn1
  ankle_rr_AxisTransform/LConn1 -- ankle_rr_OriginTransform/RConn1
  knee_rr_AxisInvTransform/RConn1 -- F/RConn1

== matlab function husky_sim - Copy/Husky_simulator/sign_conversion1 ==
  data: q_des input size=12; q_des_sign_converted output size=12
% Changes sign on angles to keep with robot sign convention
%
%   Positive input results in
%   hip frontal - rotate CW (away from body)
%   hip sagittal - rotate CW (rotate leg forward relative to initial position)
%   knee - rotate CW (extension)
%
% Input: q_des  desired input angles
%        angles must be in the following order:
%   q_FR_HF
%   q_FR_HS
%   q_FR_K
%   q_FL_HF
%   q_FL_HS
%   q_FL_K
%   q_BR_HF 
%   q_BR_HS
%   q_BR_K 
%   q_BL_HF 
%   q_BL_HS 
%   q_BL_K 
%
%   Where, FR, FL, BR, BL refers to front right, front left, back right,
%          and back left leg respectively
%       HF, HS, K refers to hip frontal, hip sagittal and knee joints
%       respectively
%
% Output: sign corrected desired angles in the same order as above
%
% By Pravin Dangol, 12-30-19, Boston MA
%
function q_des_sign_converted = func_sign_conversion(q_des)

q_des_sign_converted = q_des;

q_des_sign_converted([2:5,9:11]) = -q_des([2:5,9:11]);

== matlab function husky_sim - Copy/Foot placement/MATLAB Function ==
  data: impact input; pair1_on_ground output; pair2_on_ground output
function [pair1_on_ground, pair2_on_ground] = func_leg_contact(impact)

if impact([1,4]) == 1
    pair1_on_ground = 1;
else
    pair1_on_ground = 0;
end

if impact([2,3]) == 1
    pair2_on_ground = 1;
else
    pair2_on_ground = 0;
end

end

== stateflow chart husky_sim - Copy/Foot placement/Chart ==
  state Phase2
    entry:
    del_pf = [0,0,0, 0,0,z_max,...
    0,0,z_max,  0,0,0];
  state Start
  state Phase1
    entry:
    del_pf = [0,0,z_max, 0,0,0,...
    0,0,0,  0,0,z_max];
  state Phase3
    entry:
    del_pf = [0,0,0, 0,0,0,...
    0,0,0,  0,0,0];
  Phase1 -> Phase2 [order 1] : [pair2_on_ground==1]
  Start -> Phase1 : [pair1_on_ground==1]
  (default) -> Start
  Phase2 -> Phase1 [order 1] : [pair1_on_ground==1]
  Phase1 -> Phase3 [order 2] : [start==0]
  Phase2 -> Phase3 [order 2] : [start==0]
  data: pair1_on_ground input; pair2_on_ground input; start input; z_max input; del_pf output

== matlab function husky_sim - Copy/Foot placement/husky_IK ==
  data: p_des input; q_des output; p_hf input; leg_params parameter
% Obtain leg angles [q_hf, q_hs, q_k] (in rads) from desired feet end  
%   cartesian coordinates for one leg
%
% Inputs: p_end_des = [x_des; y_des; z_des] desired coordinates of feet end 
%           reative to reference frame (located at frontal hip motor)
%         p_hf = [x0; y0; z0] body reference frame at hip frontal motor
%         leg_params = [l_offset l1 l2 l3,...
%           q_hf_offset q_hs_offset q_k_offset] leg lengths and angle
%           offsets (in rads) - see notes
% 
% Prameters: 
%   leg_params - parameters needed for computing FK or IK in each leg
%       [l_hip_offset, l1, l2, l3, q_hf_offset, q_hs_offset, q_k_offset]
%       (see notes)
%
% Output: q_des =  (12x1)[q_HF, q_HS, q_K] hip frontal, hip sagittal and knee
%  angles (in rads) based on IK in the following order
%       [q_FR_HF; q_FR_HS; q_FR_K;
%       q_FL_HF; q_FL_HS; q_FL_K
%       q_BR_HF; q_BR_HS; q_BR_K
%       q_BL_HF; q_BL_HS; q_BL_K]
%
% NOTES: 
%
% by Pravin Dangol, Boston, MA, 12-05-19
function q_des = func_IK_Husky(p_des, p_hf, leg_params)

p_hf_FR = p_hf(1:3);
p_hf_FL = p_hf(4:6);
p_hf_BR = p_hf(7:9);
p_hf_BL = p_hf(10:12);

p_des_FR = p_des(1:3);
p_des_FL = p_des(4:6);
p_des_BR = p_des(7:9);
p_des_BL = p_des(10:12);


q_FR_des = func_IK_right_leg(p_des_FR, p_hf_FR, leg_params);

q_BR_des = func_IK_right_leg(p_des_BR, p_hf_BR, leg_params);

% Left leg IK, different function used to stay consistent with chosen 
% sign convention, i.e. positive q_hf is leg rotating outwards, which is
% coutner clockwise, as apposed to clockwise for right legs
q_FL_des = func_IK_left_leg(p_des_FL, p_hf_FL, leg_params);

q_BL_des = func_IK_left_leg(p_des_BL, p_hf_BL, leg_params);


q_des = [q_FR_des; q_FL_des; q_BR_des; q_BL_des];


end

% inverse kinematics
function qd = func_IK_right_leg(p_des, p_hf, leg_params)

l_offset = leg_params(1);
l1 = leg_params(2);
l2 = leg_params(3);
l3 = leg_params(4);
q_hf_offset = leg_params(5);
q_hs_offset  = leg_params(6);
q_k_offset = leg_params(7);

% Length and parameters from the 2D leg plane, see notes
k = l1/l3;
l5 = l_offset;
l9 = sqrt((p_des(1)-p_hf(1))^2);
l6 = sqrt((p_des(3)-p_hf(3))^2+(p_des(2)-p_hf(2))^2);

% saturate lowest values to 0 before passing to sqrt()
l6_l5 = max(l6^2-l5^2,0);

l8 = sqrt(l6_l5);
lv = sqrt(l9^2+l8^2);
lv2 = lv/(k+1);
% lv1 = lv2*k;
l2a = l2/(k+1);
% l2b = l2a*k;

% Values from triangle ABC formed by the feet end, hip frontal and hip
% sagittal (see notes)
[~,q_k_prime,~] = func_triangle_angles(l2a,lv2,l3);

% calculate q_hf
beta2 = atan2(l8,l5);
temp2 = -(p_des(2)-p_hf(2))/sqrt(l5^2+l8^2);

% Saturate inputs to asin, so there is no complex output
temp2 = min(max(temp2, -1), 1);

q_hf_prime = pi-asin(temp2)-beta2;

% Note: need to keep q_hf_prime within 0 and pi inorder to avoid 1/0
%   Add saturation below

% calculate q_hs
l8_actual =  -(l5*cos(q_hf_prime) + (p_des(3)-p_hf(3)))/(sin(q_hf_prime));
% l8_actual = -(l5*cos(q_hf_prime) + (p_des(3)-p_hf(3)))/(sin(q_hf_prime));
l9_actual = (p_des(1)-p_hf(1));
beta1 = atan2(l8_actual,l9_actual);
temp1 = ((l1+l3)-l2*cos(q_k_prime))/sqrt(l8_actual^2+l9_actual^2);

% Saturate inputs to asin, so there is no complex output
temp1 = min(max(temp1, -1), 1);

q_hs_prime = pi-asin(temp1)-beta1;


% Subtract offsets from angles so 0 angle corresponds with the zero/startup 
%  configuration of husky
q_hf = q_hf_offset - q_hf_prime ;
q_hs = q_hs_prime - q_hs_offset;
q_k = q_k_prime - q_k_offset;

qd = [q_hf; q_hs; q_k];

end

function qd = func_IK_left_leg(p_des, p_hf, leg_params)

l_offset = -leg_params(1);
l1 = leg_params(2);
l2 = leg_params(3);
l3 = leg_params(4);
q_hf_offset = leg_params(5);
q_hs_offset  = leg_params(6);
q_k_offset = leg_params(7);

% Length and parameters from the 2D leg plane, see notes
k = l1/l3;
l5 = l_offset;
l9 = sqrt((p_des(1)-p_hf(1))^2);
l6 = sqrt((p_des(3)-p_hf(3))^2+(p_des(2)-p_hf(2))^2);

% saturate lowest values to 0 before passing to sqrt()
l6_l5 = max(l6^2-l5^2,0);

l8 = sqrt(l6_l5);
lv = sqrt(l9^2+l8^2);
lv2 = lv/(k+1);
% lv1 = lv2*k;
l2a = l2/(k+1);
% l2b = l2a*k;

% Values from triangle ABC formed by the feet end, hip frontal and hip
% sagittal (see notes)
[~,q_k_prime,~] = func_triangle_angles(l2a,lv2,l3);

% calculate q_hf
beta2 = atan2(l8,l5);
temp2 = -(p_des(2)-p_hf(2))/sqrt(l5^2+l8^2);

% Saturate inputs to asin, so there is no complex output
temp2 = min(max(temp2, -1), 1);

q_hf_prime = pi-asin(temp2)-beta2;

% Note: need to keep q_hf_prime within 0 and pi inorder to avoid 1/0
%   Add saturation below

% calculate q_hs
l8_actual =  -(l5*cos(q_hf_prime) + (p_des(3)-p_hf(3)))/(sin(q_hf_prime));
% l8_actual = -(l5*cos(q_hf_prime) + (p_des(3)-p_hf(3)))/(sin(q_hf_prime));
l9_actual = (p_des(1)-p_hf(1));
beta1 = atan2(l8_actual,l9_actual);
temp1 = ((l1+l3)-l2*cos(q_k_prime))/sqrt(l8_actual^2+l9_actual^2);

% Saturate inputs to asin, so there is no complex output
temp1 = min(max(temp1, -1), 1);

q_hs_prime = pi-asin(temp1)-beta1;


% Subtract offsets from angles so 0 angle corresponds with the zero/startup 
%  configuration of husky
q_hf = q_hf_offset - q_hf_prime ;
q_hs = q_hs_prime - q_hs_offset;
q_k = q_k_prime - q_k_offset;

% NOTE: q_hf should be negative due to change in sign convention for leg leg,
% compared to right
qd = [-q_hf; q_hs; q_k];


end

% use trigonometry to obtain the angles of a triangle 
%
% input:
%   lines with dims a,b and c
%
% output:
%   theta1: angle between a and c
%   theta2: angle between c and b
%   theta3: angle between b and a
%
% By Xuyang Sun
function [theta1,theta2,theta3] = func_triangle_angles(a,b,c)
c1 = func_law_of_cosine(a,b,c);
c2 = func_law_of_cosine(b,a,c);
c3 = func_law_of_cosine(c,b,a);

% Saturate inputs to acos, so there is no complex output
c1 = min(max(c1, -1), 1);
c2 = min(max(c2, -1), 1);
c3 = min(max(c3, -1), 1);

theta1 = acos(c1);
theta2 = acos(c2);
theta3 = acos(c3);
end


% obtain cos(theta) based on given the lengths of a triangle
%
% input:
%   C: dim of line in front of theta
%   A, B: dim of lines adjacent to theta
%
% output:
%   q: cos(theta)
%
% By Xuyang Sun
function q = func_law_of_cosine(C,A,B)

% if A == 0 || B == 0
%     
% end

q = (-C^2+A^2+B^2)/(2*A*B);

end

== matlab function husky_sim - Copy/Foot placement/cubic_traj_waypoints ==
  data: t input; p_end_des output; p0 input; pf input; v0 input; vf input; T_f input
function p_end_des = func_cubic_trajectory(t, p0, pf, v0, vf, T_f)

p0_FR = p0(1:3);
p0_FL = p0(4:6);
p0_BR = p0(7:9);
p0_BL = p0(10:12);

pf_FR = pf(1:3);
pf_FL = pf(4:6);
pf_BR = pf(7:9);
pf_BL = pf(10:12);

v0_FR = v0(1:3);
v0_FL = v0(4:6);
v0_BR = v0(7:9);
v0_BL = v0(10:12);

vf_FR = vf(1:3);
vf_FL = vf(4:6);
vf_BR = vf(7:9);
vf_BL = vf(10:12);

% NOTE: currently all legs must have same time to desired position
%
% Need to change this later so legs can move independently
T_f_FR = T_f(1);
T_f_FL = T_f(1);
T_f_BR = T_f(1);
T_f_BL = T_f(1);



[a0_FR,a1_FR,a2_FR,a3_FR] = func_cubic_traj_coeff(p0_FR,pf_FR,v0_FR,vf_FR, T_f_FR);

[a0_FL,a1_FL,a2_FL,a3_FL] = func_cubic_traj_coeff(p0_FL,pf_FL,v0_FL,vf_FL, T_f_FL);

[a0_BR,a1_BR,a2_BR,a3_BR] = func_cubic_traj_coeff(p0_BR,pf_BR,v0_BR,vf_BR, T_f_BR);

[a0_BL,a1_BL,a2_BL,a3_BL] = func_cubic_traj_coeff(p0_BL,pf_BL,v0_BL,vf_BL, T_f_BL);


p_end_FR = a0_FR + a1_FR.*t + a2_FR.*t^2 + a3_FR.*t^3;
p_end_FL = a0_FL + a1_FL.*t + a2_FL.*t^2 + a3_FL.*t^3;
p_end_BR = a0_BR + a1_BR.*t + a2_BR.*t^2 + a3_BR.*t^3;
p_end_BL = a0_BL + a1_BL.*t + a2_BL.*t^2 + a3_BL.*t^3;

p_end_des = [p_end_FR; p_end_FL; p_end_BR; p_end_BL];

end





% coeffs for x y z axis for 1 leg
function [a0,a1,a2,a3] = func_cubic_traj_coeff(p0,pf,v0,vf, T_f)

x0 = p0(1);
xf = pf(1);
dx0 = v0(1);
dxf = vf(1);

y0 = p0(2);
yf = pf(2);
dy0 = v0(2);
dyf = vf(2);

z0 = p0(3);
zf = pf(3);
dz0 = v0(3);
dzf = vf(3);

% Generate coefficients for cubic position trajectory in the form:
%   p = a0 + a1*t + a2*t^2 + a3*t^3
% Resulting in velocity trajectory:
%   dp = a1 + 2*a2*t + 3*a3*t^2

[a0x,a1x,a2x,a3x] = get_coeff(x0,xf,dx0,dxf, T_f);

[a0y,a1y,a2y,a3y] = get_coeff(y0,yf,dy0,dyf, T_f);

[a0z,a1z,a2z,a3z] = get_coeff(z0,zf,dz0,dzf, T_f);

a0 = [a0x; a0y; a0z];
a1 = [a1x; a1y; a1z];
a2 = [a2x; a2y; a2z];
a3 = [a3x; a3y; a3z];

end

% Generate coefficients for cubic trajectory in the form:
%   p = a0 + a1*t + a2*t^2 + a3*t^3
%   dp = a1 + 2*a2*t + 3*a3*t^2
function [a0,a1,a2,a3] = get_coeff(p0,pf,v0,vf, T_f)

a0 = p0;
a1 = v0;

A = [T_f^2 T_f^3; 2*T_f 3*T_f^2];

B = [pf - a0 - a1*T_f; vf - a1];

temp = A\B;

a2 = temp(1);
a3 = temp(2);

end
